simulink model "plant_1"  (R2024b)
settings: Solver=VariableStepAuto  StartTime=0.0  StopTime=1000  FixedStep=10e-5
settings Model: Creator=Mehmet  LastModifiedBy=mehmet
settings SolverCC: AlgebraicLoopSolver=TrustRegion
settings DataIOCC: ReturnWorkspaceOutputs=off
settings DebuggingCC: UnconnectedInputMsg=warning  UnconnectedOutputMsg=warning  UnconnectedLineMsg=warning  ArithmeticOperatorsInVariantConditions=warning
settings ModelReferenceCC: EnableRefExpFcnMdlSchedulingChecks=on
settings SFSimCC: SimUseLocalCustomCode=off  CustomCodeUndefinedFunction=UseInterfaceOnly
settings RTWCC: RTWUseLocalCustomCode=off  GPUComputeCapability=3.5

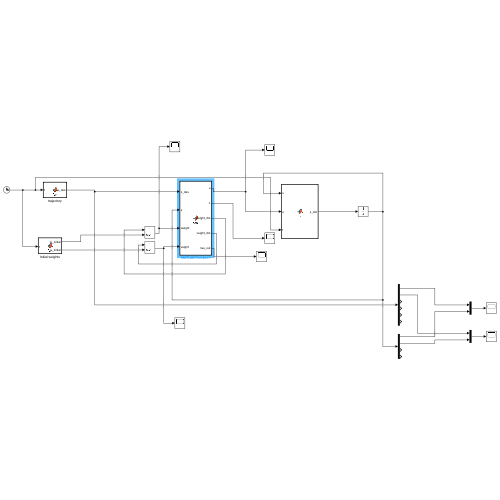
[thumbnail: Simulink's stored preview of the top-level diagram]
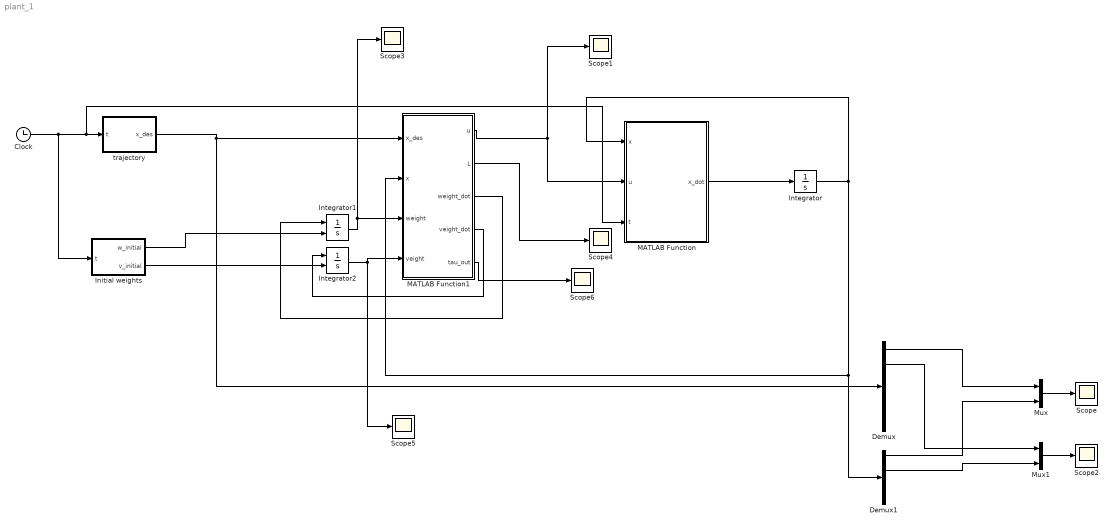
== system plant_1 ==
  Clock : Clock
  Demux : Demux  Outputs=6
  Demux1 : Demux
  Initial weights : MATLAB Function  TreatAsAtomicUnit=on
  Integrator : Integrator  InitialCondition=[0;0;0;0]
  Integrator1 : Integrator  InitialConditionSource=external  InitialCondition=[0;0]
  Integrator2 : Integrator  InitialConditionSource=external  InitialCondition=[0;0]
  MATLAB Function : MATLAB Function  TreatAsAtomicUnit=on
  MATLAB Function1 : MATLAB Function  TreatAsAtomicUnit=on
  Mux : Mux  Inputs=2
  Mux1 : Mux  Inputs=2
  Scope{,1..6} (7 alike) : Scope
  trajectory : MATLAB Function  TreatAsAtomicUnit=on
  wires:
  Clock/1 -> Initial weights/1(t), MATLAB Function/3(t), trajectory/1(t)
  trajectory/1(x_des) -> MATLAB Function1/1(x_des), Demux/1
  Demux/1 -> Mux/1
  Demux1/1 -> Mux/2
  Mux/1 -> Scope/1
  MATLAB Function/1(x_dot) -> Integrator/1
  Integrator/1 -> MATLAB Function1/2(x), Demux1/1, MATLAB Function/1(x)
  Mux1/1 -> Scope2/1
  Demux/2 -> Mux1/1
  Demux1/2 -> Mux1/2
  MATLAB Function1/3(weight_dot) -> Integrator1/1
  Integrator1/1 -> Scope3/1, MATLAB Function1/3(weight)
  MATLAB Function1/2(L) -> Scope4/1
  Initial weights/1(w_initial) -> Integrator1/2
  Integrator2/1 -> Scope5/1, MATLAB Function1/4(veight)
  MATLAB Function1/4(veight_dot) -> Integrator2/1
  Initial weights/2(v_initial) -> Integrator2/2
  MATLAB Function1/5(tau_out) -> Scope6/1
  MATLAB Function1/1(u) -> MATLAB Function/2(u), Scope1/1

== matlab function plant_1/MATLAB Function1 ==
  data: x_des input; u output; L output; x input; weight input; weight_dot output; veight input; veight_dot output; tau_out output
function [u,L,weight_dot,veight_dot,tau_out]  = fcn(x_des,x,weight,veight)

g= 9.81; % arm parameters
 
Kv = 5*eye(2); % controller parameters
lam = 1*eye(2);

% tracking errors
qd = x_des(1:2,1);
qdp = x_des(3:4,1);
qdpp = x_des(5:6,1);

e = qd - [x(1) x(2)]';
ep = qdp - [x(3) x(4)]';
r = ep + lam*e;


%%%%%%%%%%%%%%%%%%%%%%%%%%%%%%%%%%%%%%%%%%%%%%%%%%%%%%%%%%
%% MLP ideal case application
% input whole parameters
H = 5;
K = 2;
I = 14;
x_new = [x(1:4)' x_des(1:6)' e' ep'];
% x_new = [sin(x(1:4)') cos(x(1:4)')];

w = weight;
v = veight;

sigma_x = zeros(H,1);
sigma_x_dot = zeros(H,1);

Z = [w, zeros(H+1,H+1);
     zeros(I,K),v];
 
Z_f_norm = norm(Z,'fro');

Zb = 1;

Kz = eye(2);

v_t = -Kz*(Z_f_norm + Zb)*r;




%%%%%%%%%%%%%%%%%%%%%%%%%%%%%%%%%%%%%%%%%%%%%%%%%%%%%%%%%%%%%%%%%%%%%%%%%%%
% output function
for h = 1 : 1 : H
    in_out = 0;
    
    for i = 1 : 1 : length(x_new)

        in_out = in_out + v(i,h)*x_new(1,i);

    end
    
    sigma_x(h,1) = 1/(1 + exp(-in_out));
    sigma_x_dot(h,1) = sigma_x(h,1)*(1 - sigma_x(h,1));
    
end

tau = zeros(K,1);

sigma_x_new = [sigma_x;1];
sigma_x_dot_new = [sigma_x_dot;0];

for k = 1 : 1 : K
   
    cont_in = 0;
    
    for h = 1 : 1 : H + 1
        
        cont_in = cont_in + w(h,k)*sigma_x_new(h,1);
        
    end
    
    tau(k) = cont_in;
    
end

% output function
%%%%%%%%%%%%%%%%%%%%%%%%%%%%%%%%%%%%%%%%%%%%%%%%%%%%%%%%%%%%%%%%%%%%%%%%%%%

%%%%%%%%%%%%%%%%%%%%%%%%%%%%%%%%%%%%%%%%%%%%%%%%%%%%%%%%%%%%%%%%%%%%%%%%%%%
%% training function

w_dot = zeros(size(w));
v_dot = zeros(size(v));

% learning rate
F = 1;
G = 1;
kappa = 0.01;

norm_r = norm(r);

for k = 1 : 1 : K
    
    for h = 1 : 1 : H + 1
   
        %w_dot(h,k) = F*sigma_x_new(h,1)*r(k) - F*sigma_x_dot_new(h,1)*x_new(1,:)*v(:,h)*r(k) - kappa*F*norm_r*w(h,k);
        w_dot(h,k) = F*sigma_x_new(h,1)*r(k) - kappa*F*norm_r*w(h,k);
        
    end
%     
%     w_dot(H + 1,k) = F*sigma_x_new(H + 1,1)*r(k) - kappa*F*norm_r*w(H + 1,k);

end

for h = 1 : 1 : H + 1
    
    for i = 1 : 1 : I
   
        v_dot(i,h) = G*norm_r*x_new(1,i)*sigma_x_new(h,1) - kappa*G*norm_r*v(i,h);
        
        %v_dot(i,h) = G*x_new(1,i)*(sigma_x_dot_new(h,1)*w(h,:)*r) - kappa*G*norm_r*v(i,h);
%        v_dot(i,h) = G*x_new(1,i)*(sigma_x_dot(h,1)*r'*w(h,:)');      
         
    end
    
    
end


%% training function
%%%%%%%%%%%%%%%%%%%%%%%%%%%%%%%%%%%%%%%%%%%%%%%%%%%%%%%%%%%%%%%%%%%%%%%%%%%


%% MLP ideal case application
%%%%%%%%%%%%%%%%%%%%%%%%%%%%%%%%%%%%%%%%%%%%%%%%%%%%%%%%%%

weight_dot = w_dot;
veight_dot = v_dot;

u = tau + Kv*r - v_t;

tau_out = tau;

L = 1/2*r'*r;


end

== matlab function plant_1/MATLAB Function ==
  data: x input; u input; x_dot output; t input
function x_dot = fcn(x,u,t)

m1 = 1.7 + sin(2*pi*t); 
m2 = 1.1 + cos(2*pi*t); 
a1 = 2.3; 
a2 = 1.3; 
g = 9.81;   

% % arm parameters
% m1 = 0.7; 
% m2 = 2.1; 
% a1 = 2.3; 
% a2 = 0.3; 
% g = 9.81;   



% inertia M(q) and nonlinear terms N(q,qdot)
M11= (m1 + m2)*a1^2 + m2*a2^2 + 2*m2*a1*a2*cos(x(2)) ;
M12= m2*a2^2 + m2*a1*a2*cos(x(2)) ;
M22= m2*a2^2 ;
N1= -m2*a1*a2*(2*x(3)*x(4) + x(4)^2)*sin(x(2)) ;
N1= N1 + (m1 + m2)*g*a1*cos(x(1)) + m2*g*a2*cos(x(1) + x(2));
N2= m2*a1*a2*x(3)^2*sin(x(2)) + m2*g*a2*cos(x(1) + x(2)) ;

% Inversion of M(q) (for large values of n, use least-squares)
det= M11*M22 - M12*M12 ;
MI11= M22/det ;
MI12= -M12/det ;
MI22= M11/det ;

tau = zeros(2,1);

tau = u;
%% control input
tau1 = tau(1,1);
tau2 = tau(2,1);

q = zeros(4,1);

q(1) = x(3);
q(2) = x(4);
q(3) = MI11*(-N1 + tau1) + MI12*(-N2 + tau2);
q(4) = MI12*(-N1 + tau1) + MI22*(-N2 + tau2);

x_dot = q;

end

== matlab function plant_1/trajectory ==
  data: t input; x_des output
function x_des = fcn(t)

% compute desired trajectory
period= 2 ; amp1= 1 ; amp2= 1 ;
fact= 2*pi/period;
sinf= sin(fact*t);
cosf= cos(fact*t);
qd= [amp1*sinf amp2*cosf];
qdp= fact*[amp1*cosf -amp2*sinf];
qdpp= -fact^2*qd;

x_des = [qd qdp qdpp]';

end

== matlab function plant_1/Initial weights ==
  data: t input; w_initial output; v_initial output
function [w_initial,v_initial]= fcn(t)

H = 5;
K = 2;
I = 14;

v = zeros(I,H+1);
w = zeros(H+1,K);

w_initial = w;
v_initial = v;


end
